simulink model "spacecraft4_5"  (R2019b)
settings: Solver=VariableStepAuto  StartTime=0.0  StopTime=10.0  RelTol=1e-3
values from neighbouring files (symbols this model uses):
  C = plot(t,w,'g')    [Project1.m]    (also in Project2.m; SIR_model.m = 0.5)
undefined symbols (not defined in the file or in its folder): Angle, Axis, K, sysKF
libraries: vrlib x6, robotcorelib x1
settings Model: Creator=Tesla  LastModifiedBy=Tesla

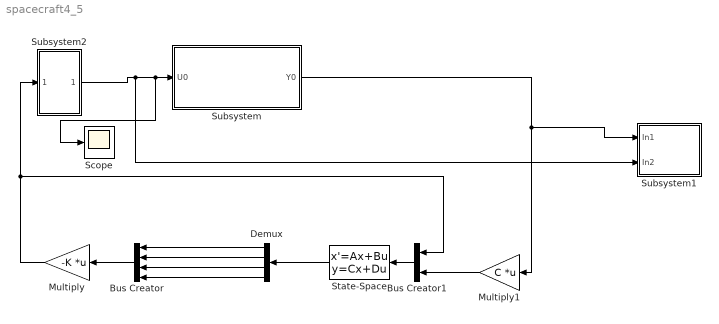
== system spacecraft4_5 ==
  Bus Creator : BusCreator  Inputs=4
  Bus Creator1 : BusCreator  Inputs=2
  Demux : Demux
  Multiply : Gain  Gain=-K  Multiplication=Matrix(K*u) (u vector)
  Multiply1 : Gain  Gain=C  Multiplication=Matrix(K*u) (u vector)
  Scope : Scope
  State-Space : StateSpace  A=sysKF.a  B=sysKF.b  C=sysKF.c  D=sysKF.d  InitialCondition=[-5 0 0 0]
  Subsystem : Subsystem
  Subsystem1 : Subsystem
  Subsystem2 : Subsystem
  wires:
  Demux/3 -> Bus Creator/3
  Demux/4 -> Bus Creator/4
  Demux/2 -> Bus Creator/2
  Demux/1 -> Bus Creator/1
  Bus Creator/1 -> Multiply/1
  State-Space/1 -> Demux/1
  Subsystem2/1(Actuator response) -> Subsystem1/2(In2), Scope/1, Subsystem/1(U0)
  Subsystem/1(Y0) -> Subsystem1/1(In1), Multiply1/1
  Multiply1/1 -> Bus Creator1/2
  Multiply/1 -> Subsystem2/1(Actuator signal), Bus Creator1/1
  Bus Creator1/1 -> State-Space/1

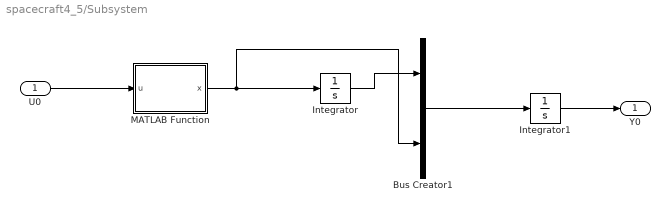
== system spacecraft4_5/Subsystem ==
  U0 : Inport
  Bus Creator1 : BusCreator  Inputs=2
  Integrator : Integrator
  Integrator1 : Integrator
  MATLAB Function : MATLAB Function  TreatAsAtomicUnit=on
  Y0 : Outport
  wires:
  MATLAB Function/1(x) -> Bus Creator1/2, Integrator/1
  U0/1 -> MATLAB Function/1(u)
  Bus Creator1/1 -> Integrator1/1
  Integrator/1 -> Bus Creator1/1
  Integrator1/1 -> Y0/1

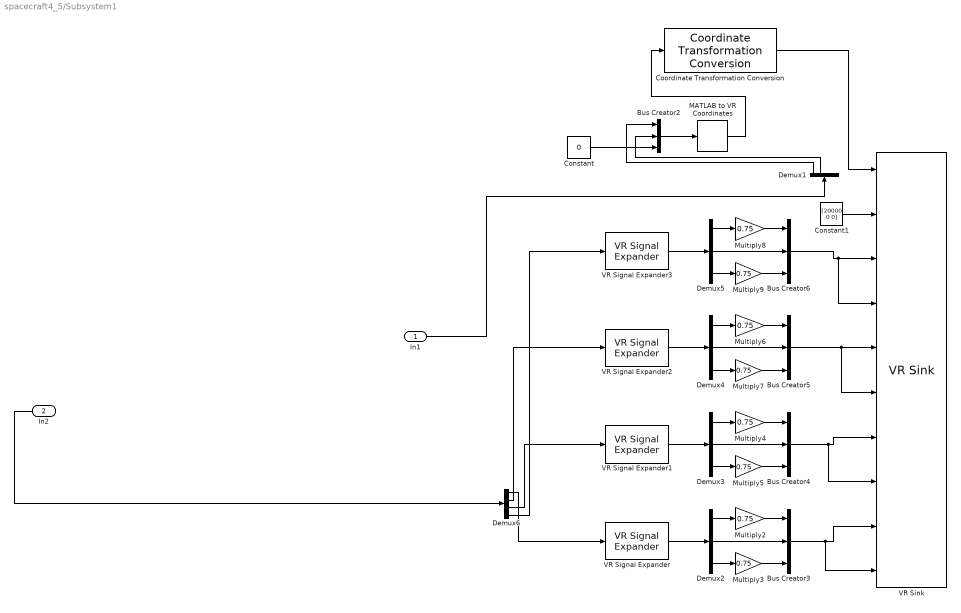
== system spacecraft4_5/Subsystem1 ==
  In1 : Inport
  In2 : Inport  Port=2
  Bus Creator{2..6} (5 alike) : BusCreator  Inputs=3
  Constant : Constant  Value=0
  Constant1 : Constant  Value=[20000 0 0]
  Coordinate Transformation Conversion : robotcorelib/Coordinate Transformation Conversion  InputRepresentation=Euler Angles  InputEulerSequence=XYZ  ShowTrVecInputPort=on  OutputRepresentation=Axis-Angle  OutputEulerSequence=ZYX  ShowTrVecOutputPort=on  SimulateUsing=Interpreted execution
      settings: SourceProductBaseCode=RO
  Demux1 : Demux
  Demux{2..5} (4 alike) : Demux  Outputs=3
  Demux6 : Demux
  MATLAB to VR Coordinates : vrlib/Utilities/MATLAB to VR Coordinates
      settings: SourceProductName=Simulink  SourceProductBaseCode=SL
  Multiply{2..9} (8 alike) : Gain  Gain=0.75
  VR Signal Expander{,1..3} (4 alike) : vrlib/VR Signal Expander  outwidth=3  outidx=[1 2 3]
      settings: SourceProductName=Simulink
  VR Sink : vrlib/VR Sink  InstantiateOnLoad=on  SampleTime=0.02  ViewEnable=on  RemoteChange=off  RemoteView=off  FieldsWritten=MB.rotation.4.1.1.double#MB.translation.3.1.1.double#Flame1.scale.3.1.1.double#Flame2.scale.3.1.1.double#Flame3.scale.3.1.1.double#Flame4.scale.3.1.1.double#Flame5.scale.3.1.1.double#Flame6.scale.3.1.1.double#Flame7.scale.3.1.1.double#Flame8.scale.3.1.1.double  WorldFileName=control systems stuff\lander vehicle\spacecraft4.wrl  AutoView=on  VideoDimensions=[500 700]  AllowVariableSize=off  FigureProperties="{'Position', 'Name', 'Viewpoint', 'CameraBound', 'CameraDirection', 'CameraPosition', 'CameraUpVector', 'ZoomFactor', 'Antialiasing', 'Headlight', 'Lighting', 'NavPanel', 'Sound', 'StatusBar', 'Stereo3D', 'Stereo3DCameraOffset', 'Stereo3DHIT', 'ToolBar', 'Textures', 'Transparency', 'Triad', 'Wireframe', 'NavZones', 'NavMode', 'NavSpeed', 'CaptureFileFormat', 'CaptureFileName', 'Record2DCompressMethod', 'Record2DCompressQuality', 'Record2D', 'Record2DFileName', 'Record2DFPS'; [5.0000000000000000e+00   9.2000000000000000e+01   5.7600000000000000e+02   3.5000000000000000e+02], '', '_untitled_1', 'on', [0.0000000000000000e+00   0.0000000000000000e+00  -1.0000000000000000e+00], [0.0000000000000000e+00   0.0000000000000000e+00   0.0000000000000000e+00], [0.0000000000000000e+00   1.0000000000000000e+00   0.0000000000000000e+00], [1.0000000000000000e+00], 'off', 'on', 'on', 'halfbar', 'on', 'on', 'off', [1.0000000149011612e-01], [0.0000000000000000e+00], 'on', 'on', 'on', 'none', 'off', 'off', 'fly', 'normal', 'tif', '%f_anim_%n.tif', 'auto', [7.5000000000000000e+01], 'off', '%f_anim_%n.avi', 'auto'}"
      settings: SourceProductName=Simulink
  wires:
  Demux6/3 -> VR Signal Expander1/1
  Demux5/1 -> Multiply8/1
  Demux6/1 -> VR Signal Expander/1
  Demux2/1 -> Multiply2/1
  Multiply3/1 -> Bus Creator3/3
  VR Signal Expander1/1 -> Demux3/1
  Demux4/3 -> Multiply7/1
  Multiply9/1 -> Bus Creator6/3
  Demux6/2 -> VR Signal Expander2/1
  Demux2/2 -> Bus Creator3/2
  Demux5/3 -> Multiply9/1
  Multiply7/1 -> Bus Creator5/3
  Bus Creator2/1 -> MATLAB to VR Coordinates/1
  MATLAB to VR Coordinates/1 -> Coordinate Transformation Conversion/1
  Demux3/1 -> Multiply4/1
  Demux1/2 -> Bus Creator2/2
  Demux3/3 -> Multiply5/1
  Demux4/1 -> Multiply6/1
  Multiply8/1 -> Bus Creator6/1
  Multiply2/1 -> Bus Creator3/1
  In2/1 -> Demux6/1
  Multiply4/1 -> Bus Creator4/1
  Demux5/2 -> Bus Creator6/2
  Demux3/2 -> Bus Creator4/2
  Demux2/3 -> Multiply3/1
  Multiply6/1 -> Bus Creator5/1
  Demux4/2 -> Bus Creator5/2
  VR Signal Expander3/1 -> Demux5/1
  VR Signal Expander/1 -> Demux2/1
  Constant/1 -> Bus Creator2/3
  Multiply5/1 -> Bus Creator4/3
  VR Signal Expander2/1 -> Demux4/1
  Demux1/1 -> Bus Creator2/1
  In1/1 -> Demux1/1
  Demux6/4 -> VR Signal Expander3/1
  Coordinate Transformation Conversion/1 -> VR Sink/1
  Bus Creator6/1 -> VR Sink/4, VR Sink/3
  Bus Creator5/1 -> VR Sink/6, VR Sink/5
  Bus Creator4/1 -> VR Sink/8, VR Sink/7
  Bus Creator3/1 -> VR Sink/10, VR Sink/9
  Constant1/1 -> VR Sink/2

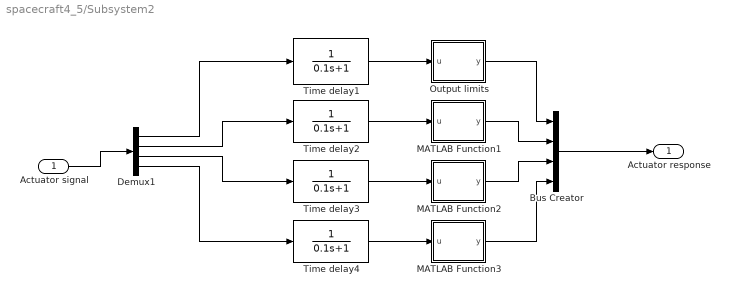
== system spacecraft4_5/Subsystem2 ==
  Actuator signal : Inport
  Bus Creator : BusCreator  Inputs=4
  Demux1 : Demux
  MATLAB Function1 : MATLAB Function  TreatAsAtomicUnit=on
  MATLAB Function2 : MATLAB Function  TreatAsAtomicUnit=on
  MATLAB Function3 : MATLAB Function  TreatAsAtomicUnit=on
  Output limits : MATLAB Function  TreatAsAtomicUnit=on
  "Time delay1 " : TransferFcn  Denominator=[0.1 1]
  Time delay2 : TransferFcn  Denominator=[0.1 1]
  Time delay3 : TransferFcn  Denominator=[0.1 1]
  Time delay4 : TransferFcn  Denominator=[0.1 1]
  Actuator response : Outport
  wires:
  Demux1/1 -> "Time delay1 "/1
  Actuator signal/1 -> Demux1/1
  Demux1/2 -> Time delay2/1
  Demux1/3 -> Time delay3/1
  Demux1/4 -> Time delay4/1
  "Time delay1 "/1 -> Output limits/1(u)
  Time delay2/1 -> MATLAB Function1/1(u)
  Bus Creator/1 -> Actuator response/1
  Output limits/1(y) -> Bus Creator/1
  MATLAB Function1/1(y) -> Bus Creator/2
  Time delay3/1 -> MATLAB Function2/1(u)
  MATLAB Function2/1(y) -> Bus Creator/3
  Time delay4/1 -> MATLAB Function3/1(u)
  MATLAB Function3/1(y) -> Bus Creator/4

== matlab function spacecraft4_5/Subsystem2/Output limits ==
  data: u input; y output
function y = fcn(u)

if u < 0;
    y = 0;
else if u > 2
    y = 2;
    else
    y = u;
        
end
end

== matlab function spacecraft4_5/Subsystem/MATLAB Function ==
  data: u input; x output
function x = fcn(u)

x = [0 0];
    
    
d = 1;
Ix = 1.5;
Iy = Ix;

F1 = u(1);
F2 = u(2);
F3 = u(3);
F4 = u(4);

theta_2dot = d*(F2-F4)/Ix
phi_2dot = d*(F1-F3)/Iy



x(1) = theta_2dot;
x(2) = phi_2dot;



end

== matlab function spacecraft4_5/Subsystem2/MATLAB Function1 ==
  data: u input; y output
function y = fcn(u)

if u < 0;
    y = 0;
else if u > 2
    y = 2;
    else
    y = u;
        
end
end

== matlab function spacecraft4_5/Subsystem2/MATLAB Function2 ==
  data: u input; y output
function y = fcn(u)

if u < 0;
    y = 0;
else if u > 2
    y = 2;
    else
    y = u;
        
end
end

== matlab function spacecraft4_5/Subsystem2/MATLAB Function3 ==
  data: u input; y output
function y = fcn(u)

if u < 0;
    y = 0;
else if u > 2
    y = 2;
    else
    y = u;
        
end
end
